simulink model "test_aero"  (R2014b)
settings: Solver=ode45  StartTime=0.0  StopTime=10.0  RelTol=1e-3
values from neighbouring files (symbols this model uses):
  TestInputs =     [unit_test_inputs.mat]
libraries: simulink x4, simulink_extras x2, csu_afm_aerodynamics_lib x1, util_frame_rotation_lib x1
settings Model: Creator=gnc  LastModifiedBy=mstewart
settings DebuggingCC: UnderspecifiedInitializationDetection=Classic  MergeDetectMultiDrivingBlocksExec=none  SolverPrmCheckMsg=none

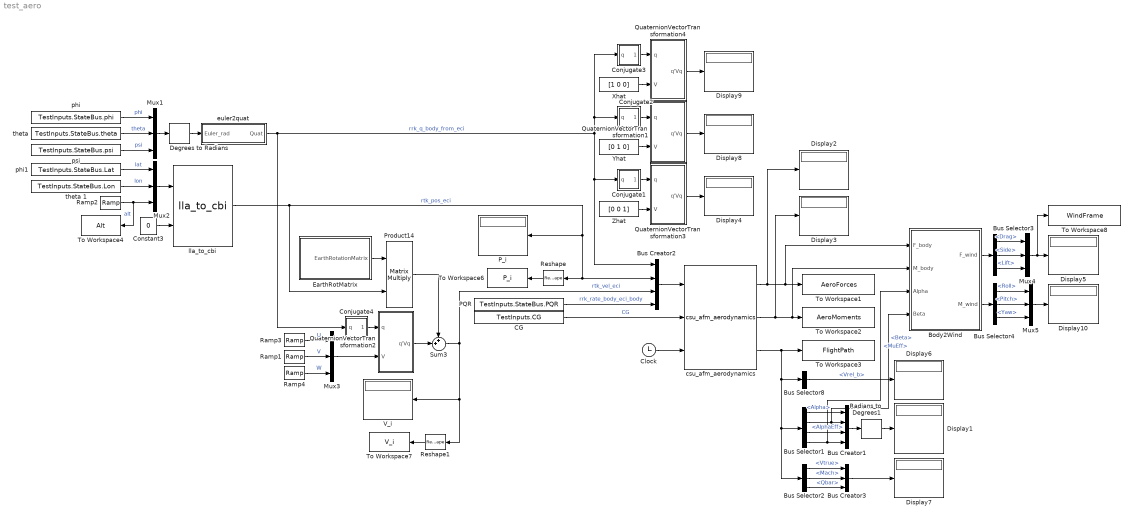
== system test_aero ==
  Body2Wind : Subsystem
  Bus Creator1 : BusCreator
  Bus Creator2 : BusCreator
  Bus Creator3 : BusCreator  Inputs=3
  Bus Selector1 : BusSelector  OutputSignals=Alpha,Beta,AlphaEff,MuEff
  Bus Selector2 : BusSelector  OutputSignals=Vtrue,Mach,Qbar
  Bus Selector3 : BusSelector  OutputSignals=Drag,Side,Lift
  Bus Selector4 : BusSelector  OutputSignals=Roll,Pitch,Yaw
  Bus Selector8 : BusSelector  OutputSignals=Vrel_b
  CG : Constant  Value=TestInputs.CG  VectorParams1D=off
  Clock : Clock
  Conjugate1 : Subsystem
  Conjugate2 : Subsystem
  Conjugate3 : Subsystem
  Conjugate4 : Subsystem
  Constant3 : Constant  Value=0
  Degrees to Radians : simulink_extras/Transformations/Degrees to Radians
  Display{1..10} (10 alike) : Display
  EarthRotMatrix : Subsystem
  Mux{1..5} (5 alike) : Mux  Inputs=3
  PQR : Constant  Value=TestInputs.StateBus.PQR  VectorParams1D=off
  P_i : Display
  Product14 : Product  Multiplication=Matrix(*)  SaturateOnIntegerOverflow=on  OutDataTypeStr=Inherit: Same as first input
  QuaternionVectorTransformation1 : Subsystem
  QuaternionVectorTransformation2 : Subsystem
  QuaternionVectorTransformation3 : Subsystem
  QuaternionVectorTransformation4 : Subsystem
  Radians to Degrees1 : simulink_extras/Transformations/Radians to Degrees
  Ramp1 : simulink/Sources/Ramp  slope=TestInputs.StateBus.Vdot  start=0  X0=TestInputs.StateBus.V
  Ramp2 : simulink/Sources/Ramp  slope=TestInputs.StateBus.AltDot  start=0  X0=TestInputs.StateBus.Alt
  Ramp3 : simulink/Sources/Ramp  slope=TestInputs.StateBus.Udot  start=0  X0=TestInputs.StateBus.U
  Ramp4 : simulink/Sources/Ramp  slope=TestInputs.StateBus.Wdot  start=0  X0=TestInputs.StateBus.W
  Reshape : Reshape
  Reshape1 : Reshape
  Sum3 : Sum  Inputs=++|
  To Workspace1 : ToWorkspace  VariableName=AeroForces  SaveFormat=Timeseries  SampleTime=-1
  To Workspace2 : ToWorkspace  VariableName=AeroMoments  SaveFormat=Timeseries  SampleTime=-1
  To Workspace3 : ToWorkspace  VariableName=FlightPath  SaveFormat=Timeseries  SampleTime=-1
  To Workspace4 : ToWorkspace  VariableName=Alt  SaveFormat=Timeseries  SampleTime=-1
  To Workspace6 : ToWorkspace  VariableName=P_i  SaveFormat=Timeseries  SampleTime=-1
  To Workspace7 : ToWorkspace  VariableName=V_i  SaveFormat=Timeseries  SampleTime=-1
  To Workspace8 : ToWorkspace  VariableName=WindFrame  SaveFormat=Timeseries  SampleTime=-1
  V_i : Display
  Xhat : Constant  Value=[1 0 0]
  Yhat : Constant  Value=[0 1 0]
  Zhat : Constant  Value=[0 0 1]
  csu_afm_aerodynamics : csu_afm_aerodynamics_lib/csu_afm_aerodynamics  SystemSampleTime=-1
  euler2quat : Subsystem
  lla_to_cbi : util_frame_rotation_lib/lla_to_cbi  a=6378137.0  flatten=1/298.257223563
  phi : Constant  Value=TestInputs.StateBus.phi  VectorParams1D=off
  phi1 : Constant  Value=TestInputs.StateBus.Lat  VectorParams1D=off
  psi : Constant  Value=TestInputs.StateBus.psi  VectorParams1D=off
  theta : Constant  Value=TestInputs.StateBus.theta  VectorParams1D=off
  theta 1 : Constant  Value=TestInputs.StateBus.Lon  VectorParams1D=off
  wires:
  Bus Creator2/1 -> csu_afm_aerodynamics/1
  Clock/1 -> csu_afm_aerodynamics/3
  CG/1 -> csu_afm_aerodynamics/2  "CG"
  csu_afm_aerodynamics/2 -> Display3/1, Body2Wind/2(M_body), To Workspace2/1
  csu_afm_aerodynamics/1 -> Display2/1, To Workspace1/1, Body2Wind/1(F_body)
  phi/1 -> Mux1/1  "phi"
  theta/1 -> Mux1/2  "theta"
  Mux1/1 -> Degrees to Radians/1
  Degrees to Radians/1 -> euler2quat/1(Euler_rad)
  psi/1 -> Mux1/3  "psi"
  euler2quat/1(Quat) -> Conjugate4/1(q), Bus Creator2/1, Conjugate1/1(q), Conjugate3/1(q), Conjugate2/1(q)  "rrk_q_body_from_eci"
  PQR/1 -> Bus Creator2/4  "rrk_rate_body_eci_body"
  Sum3/1 -> Reshape1/1, V_i/1, Bus Creator2/3  "rtk_vel_eci"
  lla_to_cbi/1 -> Product14/2, Bus Creator2/2, Reshape/1, P_i/1  "rtk_pos_eci"
  Constant3/1 -> lla_to_cbi/2
  Mux2/1 -> lla_to_cbi/1
  theta 1/1 -> Mux2/2  "lon"
  Ramp2/1 -> To Workspace4/1, Mux2/3  "alt"
  phi1/1 -> Mux2/1  "lat"
  csu_afm_aerodynamics/3 -> Bus Selector1/1, Bus Selector2/1, Bus Selector8/1, To Workspace3/1
  Zhat/1 -> QuaternionVectorTransformation3/2(V)
  QuaternionVectorTransformation3/1(q'Vq) -> Display4/1
  Conjugate1/1(q') -> QuaternionVectorTransformation3/1(q)
  Yhat/1 -> QuaternionVectorTransformation1/2(V)
  QuaternionVectorTransformation1/1(q'Vq) -> Display8/1
  Conjugate2/1(q') -> QuaternionVectorTransformation1/1(q)
  Xhat/1 -> QuaternionVectorTransformation4/2(V)
  QuaternionVectorTransformation4/1(q'Vq) -> Display9/1
  Conjugate3/1(q') -> QuaternionVectorTransformation4/1(q)
  Bus Selector8/1 -> Display6/1  "<Vrel_b>"
  Bus Selector1/4 -> Body2Wind/3(Alpha), Bus Creator1/4  "<MuEff>"
  Bus Selector1/3 -> Bus Creator1/3  "<AlphaEff>"
  Bus Selector1/2 -> Body2Wind/4(Beta), Bus Creator1/2  "<Beta>"
  Bus Selector1/1 -> Bus Creator1/1  "<Alpha>"
  Bus Creator3/1 -> Display7/1
  Ramp3/1 -> Mux3/1  "U"
  Ramp1/1 -> Mux3/2  "V"
  Mux3/1 -> QuaternionVectorTransformation2/2(V)
  Ramp4/1 -> Mux3/3  "W"
  Conjugate4/1(q') -> QuaternionVectorTransformation2/1(q)
  EarthRotMatrix/1(EarthRotationMatrix) -> Product14/1
  QuaternionVectorTransformation2/1(q'Vq) -> Sum3/2
  Product14/1 -> Sum3/1
  Reshape1/1 -> To Workspace7/1
  Reshape/1 -> To Workspace6/1
  Bus Creator1/1 -> Radians to Degrees1/1
  Radians to Degrees1/1 -> Display1/1
  Body2Wind/1(F_wind) -> Bus Selector3/1
  Mux4/1 -> To Workspace8/1, Display5/1
  Bus Selector3/1 -> Mux4/1  "<Drag>"
  Bus Selector3/2 -> Mux4/2  "<Side>"
  Bus Selector3/3 -> Mux4/3  "<Lift>"
  Bus Selector2/1 -> Bus Creator3/1  "<Vtrue>"
  Bus Selector2/2 -> Bus Creator3/2  "<Mach>"
  Bus Selector2/3 -> Bus Creator3/3  "<Qbar>"
  Body2Wind/2(M_wind) -> Bus Selector4/1
  Bus Selector4/1 -> Mux5/1  "<Roll>"
  Bus Selector4/2 -> Mux5/2  "<Pitch>"
  Bus Selector4/3 -> Mux5/3  "<Yaw>"
  Mux5/1 -> Display10/1

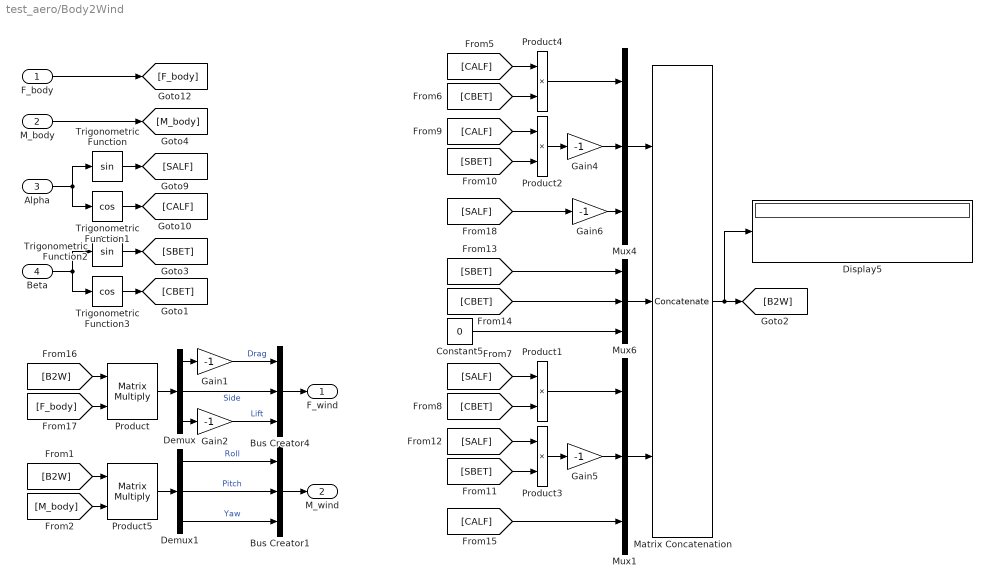
== system test_aero/Body2Wind ==
  F_body : Inport
  M_body : Inport  Port=2
  Alpha : Inport  Port=3
  Beta : Inport  Port=4
  Bus Creator1 : BusCreator  Inputs=3
  Bus Creator4 : BusCreator  Inputs=3
  Constant5 : Constant  Value=0
  Demux : Demux  Outputs=3
  Demux1 : Demux  Outputs=3
  Display5 : Display
  Gain{1..2,4..6} (5 alike) : Gain  Gain=-1  SaturateOnIntegerOverflow=on  OutDataTypeStr=Inherit: Same as input  ParamDataTypeStr=Inherit: Same as input
  Matrix Concatenation : Concatenate  NumInputs=3  Mode=Multidimensional array  ConcatenateDimension=2
  Mux1 : Mux  Inputs=3
  Mux4 : Mux  Inputs=3
  Mux6 : Mux  Inputs=3
  Product : Product  Multiplication=Matrix(*)  SaturateOnIntegerOverflow=on  OutDataTypeStr=Inherit: Same as first input
  Product{1..4} (4 alike) : Product  RndMeth=Zero
  Product5 : Product  Multiplication=Matrix(*)  SaturateOnIntegerOverflow=on  OutDataTypeStr=Inherit: Same as first input
  Trigonometric Function : Trigonometry
  Trigonometric Function1 : Trigonometry  Operator=cos
  Trigonometric Function2 : Trigonometry
  Trigonometric Function3 : Trigonometry  Operator=cos
  F_wind : Outport
  M_wind : Outport  Port=2
  wires:
  Trigonometric Function/1 -> [SALF]
  Trigonometric Function1/1 -> [CALF]
  Alpha/1 -> Trigonometric Function1/1, Trigonometric Function/1
  [B2W] -> Product/1
  [F_body] -> Product/2
  Product/1 -> Demux/1
  Demux/1 -> Gain1/1
  Demux/3 -> Gain2/1
  F_body/1 -> [F_body]
  Bus Creator4/1 -> F_wind/1
  Gain1/1 -> Bus Creator4/1  "Drag"
  Demux/2 -> Bus Creator4/2  "Side"
  Gain2/1 -> Bus Creator4/3  "Lift"
  Trigonometric Function2/1 -> [SBET]
  Trigonometric Function3/1 -> [CBET]
  Beta/1 -> Trigonometric Function3/1, Trigonometric Function2/1
  [CALF] -> Product4/1
  [CBET] -> Product4/2
  Product4/1 -> Mux4/1
  Matrix Concatenation/1 -> Display5/1, [B2W]
  Mux4/1 -> Matrix Concatenation/1
  [SALF] -> Product1/1
  [CBET] -> Product1/2
  [CALF] -> Product2/1
  [SBET] -> Product2/2
  Product2/1 -> Gain4/1
  [SALF] -> Gain6/1
  Mux6/1 -> Matrix Concatenation/2
  [SBET] -> Mux6/1
  Gain4/1 -> Mux4/2
  Gain6/1 -> Mux4/3
  Mux1/1 -> Matrix Concatenation/3
  Constant5/1 -> Mux6/3
  [CBET] -> Mux6/2
  Product1/1 -> Mux1/1
  [SALF] -> Product3/1
  [SBET] -> Product3/2
  Product3/1 -> Gain5/1
  Gain5/1 -> Mux1/2
  [CALF] -> Mux1/3
  [B2W] -> Product5/1
  [M_body] -> Product5/2
  Product5/1 -> Demux1/1
  Bus Creator1/1 -> M_wind/1
  Demux1/1 -> Bus Creator1/1  "Roll"
  Demux1/2 -> Bus Creator1/2  "Pitch"
  Demux1/3 -> Bus Creator1/3  "Yaw"
  M_body/1 -> [M_body]

== system test_aero/Conjugate1 ==
  q : Inport  PortDimensions=4
  Demux : Demux  Outputs=[3 1]
  Gain : Gain  Gain=-1  SaturateOnIntegerOverflow=on  OutDataTypeStr=Inherit: Same as input  ParamDataTypeStr=Inherit: Same as input
  Mux : Mux  Inputs=2
  q' : Outport  InitialOutput=0
  wires:
  q/1 -> Demux/1
  Demux/1 -> Gain/1  "[ q(1)  q(2)  q(3) ]"
  Gain/1 -> Mux/1
  Demux/2 -> Mux/2  "q(4)"
  Mux/1 -> q'/1

== system test_aero/Conjugate2 ==
  q : Inport  PortDimensions=4
  Demux : Demux  Outputs=[3 1]
  Gain : Gain  Gain=-1  SaturateOnIntegerOverflow=on  OutDataTypeStr=Inherit: Same as input  ParamDataTypeStr=Inherit: Same as input
  Mux : Mux  Inputs=2
  q' : Outport  InitialOutput=0
  wires:
  Mux/1 -> q'/1
  Demux/2 -> Mux/2  "q(4)"
  Gain/1 -> Mux/1
  Demux/1 -> Gain/1  "[ q(1)  q(2)  q(3) ]"
  q/1 -> Demux/1

== system test_aero/Conjugate3 ==
  q : Inport  PortDimensions=4
  Demux : Demux  Outputs=[3 1]
  Gain : Gain  Gain=-1  SaturateOnIntegerOverflow=on  OutDataTypeStr=Inherit: Same as input  ParamDataTypeStr=Inherit: Same as input
  Mux : Mux  Inputs=2
  q' : Outport  InitialOutput=0
  wires:
  Mux/1 -> q'/1
  Demux/2 -> Mux/2  "q(4)"
  Gain/1 -> Mux/1
  Demux/1 -> Gain/1  "[ q(1)  q(2)  q(3) ]"
  q/1 -> Demux/1

== system test_aero/Conjugate4 ==
  q : Inport  PortDimensions=4
  Demux : Demux  Outputs=[3 1]
  Gain : Gain  Gain=-1  SaturateOnIntegerOverflow=on  OutDataTypeStr=Inherit: Same as input  ParamDataTypeStr=Inherit: Same as input
  Mux : Mux  Inputs=2
  q' : Outport  InitialOutput=0
  wires:
  q/1 -> Demux/1
  Demux/1 -> Gain/1  "[ q(1)  q(2)  q(3) ]"
  Gain/1 -> Mux/1
  Demux/2 -> Mux/2  "q(4)"
  Mux/1 -> q'/1

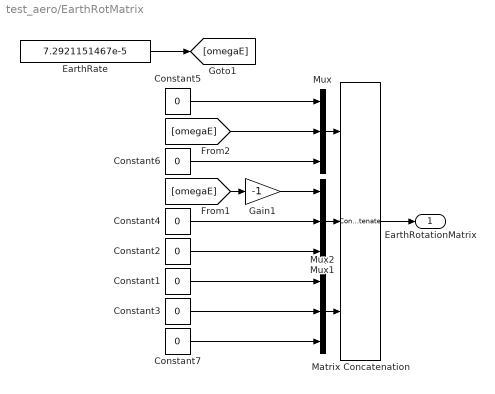
== system test_aero/EarthRotMatrix ==
  Constant{1..7} (7 alike) : Constant  Value=0
  EarthRate : Constant  Value=7.2921151467e-5
  Gain1 : Gain  Gain=-1  SaturateOnIntegerOverflow=on  OutDataTypeStr=Inherit: Same as input  ParamDataTypeStr=Inherit: Same as input
  Matrix Concatenation : Concatenate  NumInputs=3  Mode=Multidimensional array  ConcatenateDimension=2
  Mux : Mux  Inputs=3
  Mux1 : Mux  Inputs=3
  Mux2 : Mux  Inputs=3
  EarthRotationMatrix : Outport
  wires:
  [omegaE] -> Gain1/1
  Mux/1 -> Matrix Concatenation/1
  Mux1/1 -> Matrix Concatenation/2
  Gain1/1 -> Mux1/1
  Constant2/1 -> Mux1/3
  Constant1/1 -> Mux2/1
  Constant3/1 -> Mux2/2
  Constant7/1 -> Mux2/3
  Constant4/1 -> Mux1/2
  Constant6/1 -> Mux/3
  Constant5/1 -> Mux/1
  [omegaE] -> Mux/2
  EarthRate/1 -> [omegaE]
  Matrix Concatenation/1 -> EarthRotationMatrix/1
  Mux2/1 -> Matrix Concatenation/3

== system test_aero/QuaternionVectorTransformation1 ==
  q : Inport  PortDimensions=4
  V : Inport  Port=2  PortDimensions=3
  Constant : Constant  Value=0
  Mux : Mux  Inputs=2
  Quaternion Conjugate : Subsystem
  Quaternion Multiply : Subsystem
  Quaternion Multiply1 : Subsystem
  Selector : Selector  InputPortWidth=4  Indices=[1 2 3]
  q'Vq : Outport  InitialOutput=0
  wires:
  Quaternion Multiply/1(q1q2) -> Quaternion Multiply1/1(q1)
  Quaternion Conjugate/1(q') -> Quaternion Multiply/1(q1)
  Mux/1 -> Quaternion Multiply/2(q2)
  Quaternion Multiply1/1(q1q2) -> Selector/1
  q/1 -> Quaternion Conjugate/1(q), Quaternion Multiply1/2(q2)
  Constant/1 -> Mux/2
  V/1 -> Mux/1
  Selector/1 -> q'Vq/1

== system test_aero/QuaternionVectorTransformation2 ==
  q : Inport  PortDimensions=4
  V : Inport  Port=2  PortDimensions=3
  Constant : Constant  Value=0
  Mux : Mux  Inputs=2
  Quaternion Conjugate : Subsystem
  Quaternion Multiply : Subsystem
  Quaternion Multiply1 : Subsystem
  Selector : Selector  InputPortWidth=4  Indices=[1 2 3]
  q'Vq : Outport  InitialOutput=0
  wires:
  Selector/1 -> q'Vq/1
  V/1 -> Mux/1
  Constant/1 -> Mux/2
  q/1 -> Quaternion Multiply1/2(q2), Quaternion Conjugate/1(q)
  Quaternion Multiply1/1(q1q2) -> Selector/1
  Mux/1 -> Quaternion Multiply/2(q2)
  Quaternion Conjugate/1(q') -> Quaternion Multiply/1(q1)
  Quaternion Multiply/1(q1q2) -> Quaternion Multiply1/1(q1)

== system test_aero/QuaternionVectorTransformation3 ==
  q : Inport  PortDimensions=4
  V : Inport  Port=2  PortDimensions=3
  Constant : Constant  Value=0
  Mux : Mux  Inputs=2
  Quaternion Conjugate : Subsystem
  Quaternion Multiply : Subsystem
  Quaternion Multiply1 : Subsystem
  Selector : Selector  InputPortWidth=4  Indices=[1 2 3]
  q'Vq : Outport  InitialOutput=0
  wires:
  Selector/1 -> q'Vq/1
  V/1 -> Mux/1
  Constant/1 -> Mux/2
  q/1 -> Quaternion Multiply1/2(q2), Quaternion Conjugate/1(q)
  Quaternion Multiply1/1(q1q2) -> Selector/1
  Mux/1 -> Quaternion Multiply/2(q2)
  Quaternion Conjugate/1(q') -> Quaternion Multiply/1(q1)
  Quaternion Multiply/1(q1q2) -> Quaternion Multiply1/1(q1)

== system test_aero/QuaternionVectorTransformation4 ==
  q : Inport  PortDimensions=4
  V : Inport  Port=2  PortDimensions=3
  Constant : Constant  Value=0
  Mux : Mux  Inputs=2
  Quaternion Conjugate : Subsystem
  Quaternion Multiply : Subsystem
  Quaternion Multiply1 : Subsystem
  Selector : Selector  InputPortWidth=4  Indices=[1 2 3]
  q'Vq : Outport  InitialOutput=0
  wires:
  Quaternion Multiply/1(q1q2) -> Quaternion Multiply1/1(q1)
  Quaternion Conjugate/1(q') -> Quaternion Multiply/1(q1)
  Mux/1 -> Quaternion Multiply/2(q2)
  Quaternion Multiply1/1(q1q2) -> Selector/1
  q/1 -> Quaternion Conjugate/1(q), Quaternion Multiply1/2(q2)
  Constant/1 -> Mux/2
  V/1 -> Mux/1
  Selector/1 -> q'Vq/1

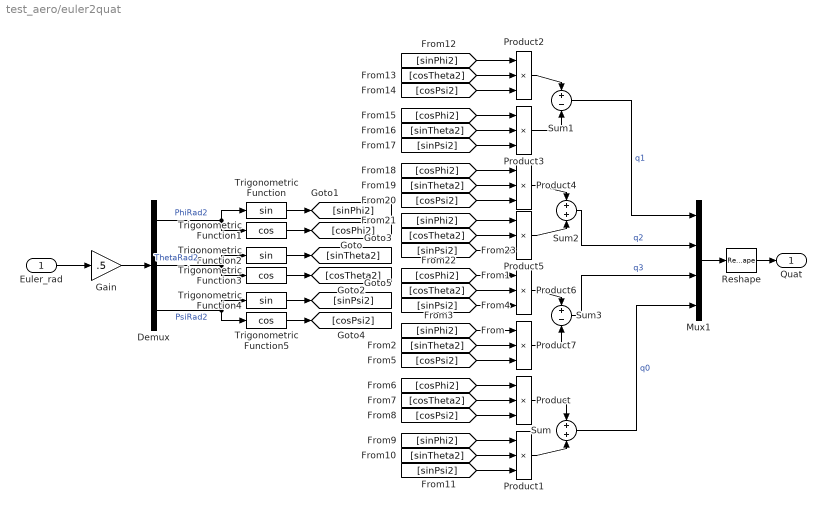
== system test_aero/euler2quat ==
  Euler_rad : Inport
  Demux : Demux  Outputs=3
  Gain : Gain  Gain=.5
  Mux1 : Mux
  Product{,1..7} (8 alike) : Product  Inputs=3  RndMeth=Zero
  Reshape : Reshape
  Sum : Sum  Inputs=+|+
  Sum1 : Sum  Inputs=+|-
  Sum2 : Sum  Inputs=+|+
  Sum3 : Sum  Inputs=+|-
  Trigonometric Function : Trigonometry
  Trigonometric Function1 : Trigonometry  Operator=cos
  Trigonometric Function2 : Trigonometry
  Trigonometric Function3 : Trigonometry  Operator=cos
  Trigonometric Function4 : Trigonometry
  Trigonometric Function5 : Trigonometry  Operator=cos
  Quat : Outport
  wires:
  Reshape/1 -> Quat/1
  Mux1/1 -> Reshape/1
  Euler_rad/1 -> Gain/1
  [cosPsi2] -> Product7/3
  [sinTheta2] -> Product7/2
  [sinPhi2] -> Product7/1
  [sinPsi2] -> Product6/3
  [cosTheta2] -> Product6/2
  [cosPhi2] -> Product6/1
  Product6/1 -> Sum3/1
  Product7/1 -> Sum3/2
  Product5/1 -> Sum2/2
  [sinPsi2] -> Product5/3
  [cosTheta2] -> Product5/2
  [sinPhi2] -> Product5/1
  Product4/1 -> Sum2/1
  [cosPsi2] -> Product4/3
  [sinTheta2] -> Product4/2
  [cosPhi2] -> Product4/1
  Product3/1 -> Sum1/2
  [sinPsi2] -> Product3/3
  [sinTheta2] -> Product3/2
  [cosPhi2] -> Product3/1
  Product2/1 -> Sum1/1
  [cosPsi2] -> Product2/3
  [cosTheta2] -> Product2/2
  [sinPhi2] -> Product2/1
  [sinPsi2] -> Product1/3
  [sinTheta2] -> Product1/2
  [sinPhi2] -> Product1/1
  Product1/1 -> Sum/2
  Product/1 -> Sum/1
  [cosPsi2] -> Product/3
  [cosTheta2] -> Product/2
  [cosPhi2] -> Product/1
  Trigonometric Function5/1 -> [cosPsi2]
  Trigonometric Function4/1 -> [sinPsi2]
  Trigonometric Function3/1 -> [cosTheta2]
  Trigonometric Function2/1 -> [sinTheta2]
  Trigonometric Function1/1 -> [cosPhi2]
  Trigonometric Function/1 -> [sinPhi2]
  Demux/3 -> Trigonometric Function5/1, Trigonometric Function4/1  "PsiRad2"
  Demux/2 -> Trigonometric Function3/1, Trigonometric Function2/1  "ThetaRad2"
  Demux/1 -> Trigonometric Function1/1, Trigonometric Function/1  "PhiRad2"
  Gain/1 -> Demux/1
  Sum1/1 -> Mux1/1  "q1"
  Sum2/1 -> Mux1/2  "q2"
  Sum3/1 -> Mux1/3  "q3"
  Sum/1 -> Mux1/4  "q0"

== system test_aero/QuaternionVectorTransformation1/Quaternion Conjugate ==
  q : Inport  PortDimensions=4
  Demux : Demux  Outputs=[3 1]
  Gain : Gain  Gain=-1  SaturateOnIntegerOverflow=on  OutDataTypeStr=Inherit: Same as input  ParamDataTypeStr=Inherit: Same as input
  Mux : Mux  Inputs=2
  q' : Outport  InitialOutput=0
  wires:
  Mux/1 -> q'/1
  Demux/2 -> Mux/2  "q(4)"
  Gain/1 -> Mux/1
  Demux/1 -> Gain/1  "[ q(1)  q(2)  q(3) ]"
  q/1 -> Demux/1

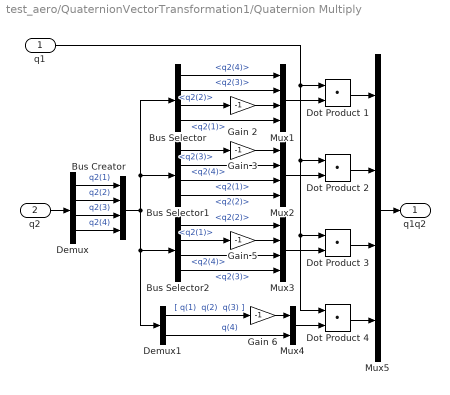
== system test_aero/QuaternionVectorTransformation1/Quaternion Multiply ==
  q1 : Inport  PortDimensions=4
  q2 : Inport  Port=2  PortDimensions=4
  Bus Creator : BusCreator
  Bus Selector : BusSelector  OutputSignals=q2(4),q2(3),q2(2),q2(1)
  Bus Selector1 : BusSelector  OutputSignals=q2(3),q2(4),q2(1),q2(2)
  Bus Selector2 : BusSelector  OutputSignals=q2(2),q2(1),q2(4),q2(3)
  Demux : Demux
  Demux1 : Demux  Outputs=[3 1]
  Dot Product {1..4} (4 alike) : DotProduct  InputSameDT=on  OutDataTypeStr=Inherit: Inherit via internal rule
  Gain {2..3,5..6} (4 alike) : Gain  Gain=-1  SaturateOnIntegerOverflow=on  OutDataTypeStr=Inherit: Same as input  ParamDataTypeStr=Inherit: Same as input
  Mux{1..3,5} (4 alike) : Mux
  Mux4 : Mux  Inputs=2
  q1q2 : Outport  InitialOutput=0
  wires:
  Demux/4 -> Bus Creator/4  "q2(4)"
  Demux/3 -> Bus Creator/3  "q2(3)"
  Demux/2 -> Bus Creator/2  "q2(2)"
  Demux/1 -> Bus Creator/1  "q2(1)"
  q2/1 -> Demux/1
  Bus Creator/1 -> Bus Selector1/1, Bus Selector/1, Bus Selector2/1, Demux1/1
  Dot Product 2/1 -> Mux5/2
  Mux5/1 -> q1q2/1
  Dot Product 4/1 -> Mux5/4
  Dot Product 3/1 -> Mux5/3
  Dot Product 1/1 -> Mux5/1
  q1/1 -> Dot Product 4/1, Dot Product 3/1, Dot Product 2/1, Dot Product 1/1
  Mux3/1 -> Dot Product 3/2
  Mux2/1 -> Dot Product 2/2
  Mux1/1 -> Dot Product 1/2
  Bus Selector2/3 -> Mux3/3  "<q2(4)>"
  Bus Selector1/2 -> Mux2/2  "<q2(4)>"
  Bus Selector/1 -> Mux1/1  "<q2(4)>"
  Bus Selector/2 -> Mux1/2  "<q2(3)>"
  Bus Selector/3 -> Gain 2/1  "<q2(2)>"
  Gain 2/1 -> Mux1/3
  Bus Selector/4 -> Mux1/4  "<q2(1)>"
  Bus Selector1/1 -> Gain 3/1  "<q2(3)>"
  Gain 3/1 -> Mux2/1
  Bus Selector1/3 -> Mux2/3  "<q2(1)>"
  Bus Selector1/4 -> Mux2/4  "<q2(2)>"
  Bus Selector2/2 -> Gain 5/1  "<q2(1)>"
  Gain 5/1 -> Mux3/2
  Bus Selector2/1 -> Mux3/1  "<q2(2)>"
  Bus Selector2/4 -> Mux3/4  "<q2(3)>"
  Mux4/1 -> Dot Product 4/2
  Demux1/1 -> Gain 6/1  "[ q(1)  q(2)  q(3) ]"
  Gain 6/1 -> Mux4/1
  Demux1/2 -> Mux4/2  "q(4)"

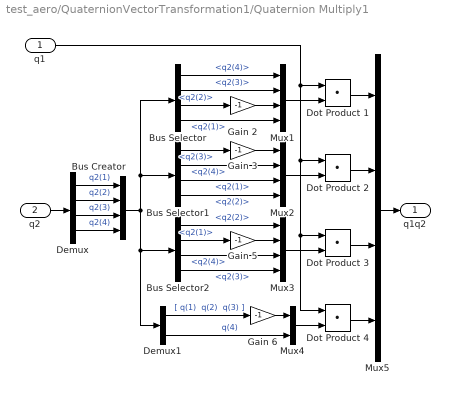
== system test_aero/QuaternionVectorTransformation1/Quaternion Multiply1 ==
  q1 : Inport  PortDimensions=4
  q2 : Inport  Port=2  PortDimensions=4
  Bus Creator : BusCreator
  Bus Selector : BusSelector  OutputSignals=q2(4),q2(3),q2(2),q2(1)
  Bus Selector1 : BusSelector  OutputSignals=q2(3),q2(4),q2(1),q2(2)
  Bus Selector2 : BusSelector  OutputSignals=q2(2),q2(1),q2(4),q2(3)
  Demux : Demux
  Demux1 : Demux  Outputs=[3 1]
  Dot Product {1..4} (4 alike) : DotProduct  InputSameDT=on  OutDataTypeStr=Inherit: Inherit via internal rule
  Gain {2..3,5..6} (4 alike) : Gain  Gain=-1  SaturateOnIntegerOverflow=on  OutDataTypeStr=Inherit: Same as input  ParamDataTypeStr=Inherit: Same as input
  Mux{1..3,5} (4 alike) : Mux
  Mux4 : Mux  Inputs=2
  q1q2 : Outport  InitialOutput=0
  wires:
  Demux/4 -> Bus Creator/4  "q2(4)"
  Demux/3 -> Bus Creator/3  "q2(3)"
  Demux/2 -> Bus Creator/2  "q2(2)"
  Demux/1 -> Bus Creator/1  "q2(1)"
  q2/1 -> Demux/1
  Bus Creator/1 -> Bus Selector1/1, Bus Selector/1, Bus Selector2/1, Demux1/1
  Dot Product 2/1 -> Mux5/2
  Mux5/1 -> q1q2/1
  Dot Product 4/1 -> Mux5/4
  Dot Product 3/1 -> Mux5/3
  Dot Product 1/1 -> Mux5/1
  q1/1 -> Dot Product 4/1, Dot Product 3/1, Dot Product 2/1, Dot Product 1/1
  Mux3/1 -> Dot Product 3/2
  Mux2/1 -> Dot Product 2/2
  Mux1/1 -> Dot Product 1/2
  Bus Selector2/3 -> Mux3/3  "<q2(4)>"
  Bus Selector1/2 -> Mux2/2  "<q2(4)>"
  Bus Selector/1 -> Mux1/1  "<q2(4)>"
  Bus Selector/2 -> Mux1/2  "<q2(3)>"
  Bus Selector/3 -> Gain 2/1  "<q2(2)>"
  Gain 2/1 -> Mux1/3
  Bus Selector/4 -> Mux1/4  "<q2(1)>"
  Bus Selector1/1 -> Gain 3/1  "<q2(3)>"
  Gain 3/1 -> Mux2/1
  Bus Selector1/3 -> Mux2/3  "<q2(1)>"
  Bus Selector1/4 -> Mux2/4  "<q2(2)>"
  Bus Selector2/2 -> Gain 5/1  "<q2(1)>"
  Gain 5/1 -> Mux3/2
  Bus Selector2/1 -> Mux3/1  "<q2(2)>"
  Bus Selector2/4 -> Mux3/4  "<q2(3)>"
  Mux4/1 -> Dot Product 4/2
  Demux1/1 -> Gain 6/1  "[ q(1)  q(2)  q(3) ]"
  Gain 6/1 -> Mux4/1
  Demux1/2 -> Mux4/2  "q(4)"

== system test_aero/QuaternionVectorTransformation2/Quaternion Conjugate ==
  q : Inport  PortDimensions=4
  Demux : Demux  Outputs=[3 1]
  Gain : Gain  Gain=-1  SaturateOnIntegerOverflow=on  OutDataTypeStr=Inherit: Same as input  ParamDataTypeStr=Inherit: Same as input
  Mux : Mux  Inputs=2
  q' : Outport  InitialOutput=0
  wires:
  q/1 -> Demux/1
  Demux/1 -> Gain/1  "[ q(1)  q(2)  q(3) ]"
  Gain/1 -> Mux/1
  Demux/2 -> Mux/2  "q(4)"
  Mux/1 -> q'/1

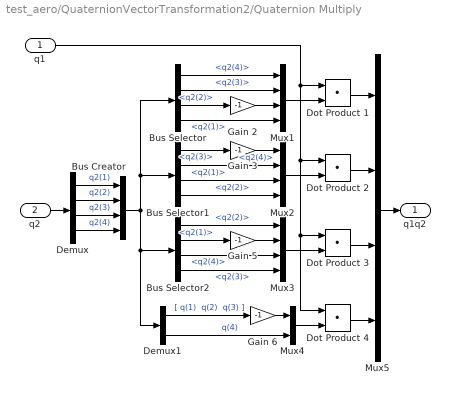
== system test_aero/QuaternionVectorTransformation2/Quaternion Multiply ==
  q1 : Inport  PortDimensions=4
  q2 : Inport  Port=2  PortDimensions=4
  Bus Creator : BusCreator
  Bus Selector : BusSelector  OutputSignals=q2(4),q2(3),q2(2),q2(1)
  Bus Selector1 : BusSelector  OutputSignals=q2(3),q2(4),q2(1),q2(2)
  Bus Selector2 : BusSelector  OutputSignals=q2(2),q2(1),q2(4),q2(3)
  Demux : Demux
  Demux1 : Demux  Outputs=[3 1]
  Dot Product {1..4} (4 alike) : DotProduct  InputSameDT=on  OutDataTypeStr=Inherit: Inherit via internal rule
  Gain {2..3,5..6} (4 alike) : Gain  Gain=-1  SaturateOnIntegerOverflow=on  OutDataTypeStr=Inherit: Same as input  ParamDataTypeStr=Inherit: Same as input
  Mux{1..3,5} (4 alike) : Mux
  Mux4 : Mux  Inputs=2
  q1q2 : Outport  InitialOutput=0
  wires:
  Demux1/2 -> Mux4/2  "q(4)"
  Gain 6/1 -> Mux4/1
  Demux1/1 -> Gain 6/1  "[ q(1)  q(2)  q(3) ]"
  Mux4/1 -> Dot Product 4/2
  Bus Selector2/4 -> Mux3/4  "<q2(3)>"
  Bus Selector2/1 -> Mux3/1  "<q2(2)>"
  Gain 5/1 -> Mux3/2
  Bus Selector2/2 -> Gain 5/1  "<q2(1)>"
  Bus Selector1/4 -> Mux2/4  "<q2(2)>"
  Bus Selector1/3 -> Mux2/3  "<q2(1)>"
  Gain 3/1 -> Mux2/1
  Bus Selector1/1 -> Gain 3/1  "<q2(3)>"
  Bus Selector/4 -> Mux1/4  "<q2(1)>"
  Gain 2/1 -> Mux1/3
  Bus Selector/3 -> Gain 2/1  "<q2(2)>"
  Bus Selector/2 -> Mux1/2  "<q2(3)>"
  Bus Selector/1 -> Mux1/1  "<q2(4)>"
  Bus Selector1/2 -> Mux2/2  "<q2(4)>"
  Bus Selector2/3 -> Mux3/3  "<q2(4)>"
  Mux1/1 -> Dot Product 1/2
  Mux2/1 -> Dot Product 2/2
  Mux3/1 -> Dot Product 3/2
  q1/1 -> Dot Product 1/1, Dot Product 2/1, Dot Product 3/1, Dot Product 4/1
  Dot Product 1/1 -> Mux5/1
  Dot Product 3/1 -> Mux5/3
  Dot Product 4/1 -> Mux5/4
  Mux5/1 -> q1q2/1
  Dot Product 2/1 -> Mux5/2
  Bus Creator/1 -> Demux1/1, Bus Selector2/1, Bus Selector/1, Bus Selector1/1
  q2/1 -> Demux/1
  Demux/1 -> Bus Creator/1  "q2(1)"
  Demux/2 -> Bus Creator/2  "q2(2)"
  Demux/3 -> Bus Creator/3  "q2(3)"
  Demux/4 -> Bus Creator/4  "q2(4)"

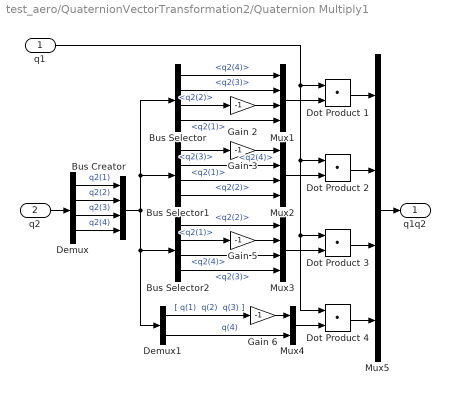
== system test_aero/QuaternionVectorTransformation2/Quaternion Multiply1 ==
  q1 : Inport  PortDimensions=4
  q2 : Inport  Port=2  PortDimensions=4
  Bus Creator : BusCreator
  Bus Selector : BusSelector  OutputSignals=q2(4),q2(3),q2(2),q2(1)
  Bus Selector1 : BusSelector  OutputSignals=q2(3),q2(4),q2(1),q2(2)
  Bus Selector2 : BusSelector  OutputSignals=q2(2),q2(1),q2(4),q2(3)
  Demux : Demux
  Demux1 : Demux  Outputs=[3 1]
  Dot Product {1..4} (4 alike) : DotProduct  InputSameDT=on  OutDataTypeStr=Inherit: Inherit via internal rule
  Gain {2..3,5..6} (4 alike) : Gain  Gain=-1  SaturateOnIntegerOverflow=on  OutDataTypeStr=Inherit: Same as input  ParamDataTypeStr=Inherit: Same as input
  Mux{1..3,5} (4 alike) : Mux
  Mux4 : Mux  Inputs=2
  q1q2 : Outport  InitialOutput=0
  wires:
  Demux1/2 -> Mux4/2  "q(4)"
  Gain 6/1 -> Mux4/1
  Demux1/1 -> Gain 6/1  "[ q(1)  q(2)  q(3) ]"
  Mux4/1 -> Dot Product 4/2
  Bus Selector2/4 -> Mux3/4  "<q2(3)>"
  Bus Selector2/1 -> Mux3/1  "<q2(2)>"
  Gain 5/1 -> Mux3/2
  Bus Selector2/2 -> Gain 5/1  "<q2(1)>"
  Bus Selector1/4 -> Mux2/4  "<q2(2)>"
  Bus Selector1/3 -> Mux2/3  "<q2(1)>"
  Gain 3/1 -> Mux2/1
  Bus Selector1/1 -> Gain 3/1  "<q2(3)>"
  Bus Selector/4 -> Mux1/4  "<q2(1)>"
  Gain 2/1 -> Mux1/3
  Bus Selector/3 -> Gain 2/1  "<q2(2)>"
  Bus Selector/2 -> Mux1/2  "<q2(3)>"
  Bus Selector/1 -> Mux1/1  "<q2(4)>"
  Bus Selector1/2 -> Mux2/2  "<q2(4)>"
  Bus Selector2/3 -> Mux3/3  "<q2(4)>"
  Mux1/1 -> Dot Product 1/2
  Mux2/1 -> Dot Product 2/2
  Mux3/1 -> Dot Product 3/2
  q1/1 -> Dot Product 1/1, Dot Product 2/1, Dot Product 3/1, Dot Product 4/1
  Dot Product 1/1 -> Mux5/1
  Dot Product 3/1 -> Mux5/3
  Dot Product 4/1 -> Mux5/4
  Mux5/1 -> q1q2/1
  Dot Product 2/1 -> Mux5/2
  Bus Creator/1 -> Demux1/1, Bus Selector2/1, Bus Selector/1, Bus Selector1/1
  q2/1 -> Demux/1
  Demux/1 -> Bus Creator/1  "q2(1)"
  Demux/2 -> Bus Creator/2  "q2(2)"
  Demux/3 -> Bus Creator/3  "q2(3)"
  Demux/4 -> Bus Creator/4  "q2(4)"

== system test_aero/QuaternionVectorTransformation3/Quaternion Conjugate ==
  q : Inport  PortDimensions=4
  Demux : Demux  Outputs=[3 1]
  Gain : Gain  Gain=-1  SaturateOnIntegerOverflow=on  OutDataTypeStr=Inherit: Same as input  ParamDataTypeStr=Inherit: Same as input
  Mux : Mux  Inputs=2
  q' : Outport  InitialOutput=0
  wires:
  q/1 -> Demux/1
  Demux/1 -> Gain/1  "[ q(1)  q(2)  q(3) ]"
  Gain/1 -> Mux/1
  Demux/2 -> Mux/2  "q(4)"
  Mux/1 -> q'/1

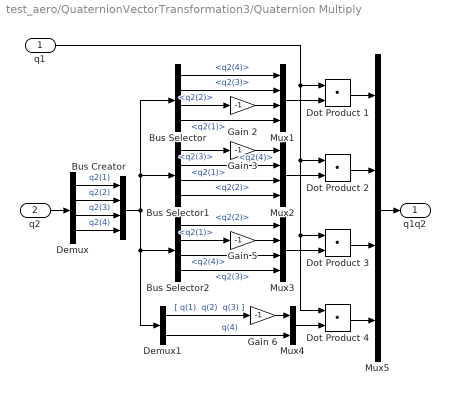
== system test_aero/QuaternionVectorTransformation3/Quaternion Multiply ==
  q1 : Inport  PortDimensions=4
  q2 : Inport  Port=2  PortDimensions=4
  Bus Creator : BusCreator
  Bus Selector : BusSelector  OutputSignals=q2(4),q2(3),q2(2),q2(1)
  Bus Selector1 : BusSelector  OutputSignals=q2(3),q2(4),q2(1),q2(2)
  Bus Selector2 : BusSelector  OutputSignals=q2(2),q2(1),q2(4),q2(3)
  Demux : Demux
  Demux1 : Demux  Outputs=[3 1]
  Dot Product {1..4} (4 alike) : DotProduct  InputSameDT=on  OutDataTypeStr=Inherit: Inherit via internal rule
  Gain {2..3,5..6} (4 alike) : Gain  Gain=-1  SaturateOnIntegerOverflow=on  OutDataTypeStr=Inherit: Same as input  ParamDataTypeStr=Inherit: Same as input
  Mux{1..3,5} (4 alike) : Mux
  Mux4 : Mux  Inputs=2
  q1q2 : Outport  InitialOutput=0
  wires:
  Demux1/2 -> Mux4/2  "q(4)"
  Gain 6/1 -> Mux4/1
  Demux1/1 -> Gain 6/1  "[ q(1)  q(2)  q(3) ]"
  Mux4/1 -> Dot Product 4/2
  Bus Selector2/4 -> Mux3/4  "<q2(3)>"
  Bus Selector2/1 -> Mux3/1  "<q2(2)>"
  Gain 5/1 -> Mux3/2
  Bus Selector2/2 -> Gain 5/1  "<q2(1)>"
  Bus Selector1/4 -> Mux2/4  "<q2(2)>"
  Bus Selector1/3 -> Mux2/3  "<q2(1)>"
  Gain 3/1 -> Mux2/1
  Bus Selector1/1 -> Gain 3/1  "<q2(3)>"
  Bus Selector/4 -> Mux1/4  "<q2(1)>"
  Gain 2/1 -> Mux1/3
  Bus Selector/3 -> Gain 2/1  "<q2(2)>"
  Bus Selector/2 -> Mux1/2  "<q2(3)>"
  Bus Selector/1 -> Mux1/1  "<q2(4)>"
  Bus Selector1/2 -> Mux2/2  "<q2(4)>"
  Bus Selector2/3 -> Mux3/3  "<q2(4)>"
  Mux1/1 -> Dot Product 1/2
  Mux2/1 -> Dot Product 2/2
  Mux3/1 -> Dot Product 3/2
  q1/1 -> Dot Product 1/1, Dot Product 2/1, Dot Product 3/1, Dot Product 4/1
  Dot Product 1/1 -> Mux5/1
  Dot Product 3/1 -> Mux5/3
  Dot Product 4/1 -> Mux5/4
  Mux5/1 -> q1q2/1
  Dot Product 2/1 -> Mux5/2
  Bus Creator/1 -> Demux1/1, Bus Selector2/1, Bus Selector/1, Bus Selector1/1
  q2/1 -> Demux/1
  Demux/1 -> Bus Creator/1  "q2(1)"
  Demux/2 -> Bus Creator/2  "q2(2)"
  Demux/3 -> Bus Creator/3  "q2(3)"
  Demux/4 -> Bus Creator/4  "q2(4)"

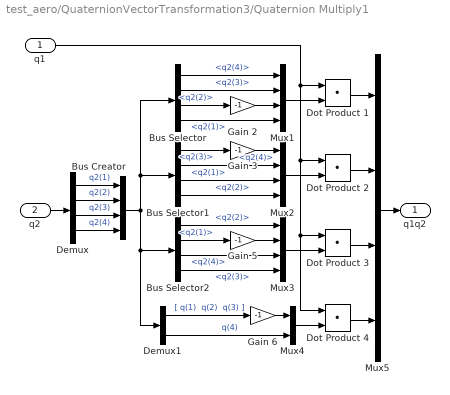
== system test_aero/QuaternionVectorTransformation3/Quaternion Multiply1 ==
  q1 : Inport  PortDimensions=4
  q2 : Inport  Port=2  PortDimensions=4
  Bus Creator : BusCreator
  Bus Selector : BusSelector  OutputSignals=q2(4),q2(3),q2(2),q2(1)
  Bus Selector1 : BusSelector  OutputSignals=q2(3),q2(4),q2(1),q2(2)
  Bus Selector2 : BusSelector  OutputSignals=q2(2),q2(1),q2(4),q2(3)
  Demux : Demux
  Demux1 : Demux  Outputs=[3 1]
  Dot Product {1..4} (4 alike) : DotProduct  InputSameDT=on  OutDataTypeStr=Inherit: Inherit via internal rule
  Gain {2..3,5..6} (4 alike) : Gain  Gain=-1  SaturateOnIntegerOverflow=on  OutDataTypeStr=Inherit: Same as input  ParamDataTypeStr=Inherit: Same as input
  Mux{1..3,5} (4 alike) : Mux
  Mux4 : Mux  Inputs=2
  q1q2 : Outport  InitialOutput=0
  wires:
  Demux1/2 -> Mux4/2  "q(4)"
  Gain 6/1 -> Mux4/1
  Demux1/1 -> Gain 6/1  "[ q(1)  q(2)  q(3) ]"
  Mux4/1 -> Dot Product 4/2
  Bus Selector2/4 -> Mux3/4  "<q2(3)>"
  Bus Selector2/1 -> Mux3/1  "<q2(2)>"
  Gain 5/1 -> Mux3/2
  Bus Selector2/2 -> Gain 5/1  "<q2(1)>"
  Bus Selector1/4 -> Mux2/4  "<q2(2)>"
  Bus Selector1/3 -> Mux2/3  "<q2(1)>"
  Gain 3/1 -> Mux2/1
  Bus Selector1/1 -> Gain 3/1  "<q2(3)>"
  Bus Selector/4 -> Mux1/4  "<q2(1)>"
  Gain 2/1 -> Mux1/3
  Bus Selector/3 -> Gain 2/1  "<q2(2)>"
  Bus Selector/2 -> Mux1/2  "<q2(3)>"
  Bus Selector/1 -> Mux1/1  "<q2(4)>"
  Bus Selector1/2 -> Mux2/2  "<q2(4)>"
  Bus Selector2/3 -> Mux3/3  "<q2(4)>"
  Mux1/1 -> Dot Product 1/2
  Mux2/1 -> Dot Product 2/2
  Mux3/1 -> Dot Product 3/2
  q1/1 -> Dot Product 1/1, Dot Product 2/1, Dot Product 3/1, Dot Product 4/1
  Dot Product 1/1 -> Mux5/1
  Dot Product 3/1 -> Mux5/3
  Dot Product 4/1 -> Mux5/4
  Mux5/1 -> q1q2/1
  Dot Product 2/1 -> Mux5/2
  Bus Creator/1 -> Demux1/1, Bus Selector2/1, Bus Selector/1, Bus Selector1/1
  q2/1 -> Demux/1
  Demux/1 -> Bus Creator/1  "q2(1)"
  Demux/2 -> Bus Creator/2  "q2(2)"
  Demux/3 -> Bus Creator/3  "q2(3)"
  Demux/4 -> Bus Creator/4  "q2(4)"

== system test_aero/QuaternionVectorTransformation4/Quaternion Conjugate ==
  q : Inport  PortDimensions=4
  Demux : Demux  Outputs=[3 1]
  Gain : Gain  Gain=-1  SaturateOnIntegerOverflow=on  OutDataTypeStr=Inherit: Same as input  ParamDataTypeStr=Inherit: Same as input
  Mux : Mux  Inputs=2
  q' : Outport  InitialOutput=0
  wires:
  Mux/1 -> q'/1
  Demux/2 -> Mux/2  "q(4)"
  Gain/1 -> Mux/1
  Demux/1 -> Gain/1  "[ q(1)  q(2)  q(3) ]"
  q/1 -> Demux/1

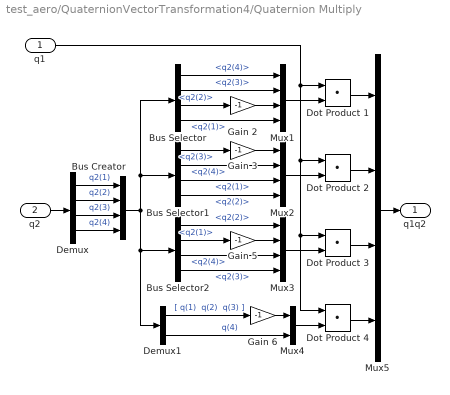
== system test_aero/QuaternionVectorTransformation4/Quaternion Multiply ==
  q1 : Inport  PortDimensions=4
  q2 : Inport  Port=2  PortDimensions=4
  Bus Creator : BusCreator
  Bus Selector : BusSelector  OutputSignals=q2(4),q2(3),q2(2),q2(1)
  Bus Selector1 : BusSelector  OutputSignals=q2(3),q2(4),q2(1),q2(2)
  Bus Selector2 : BusSelector  OutputSignals=q2(2),q2(1),q2(4),q2(3)
  Demux : Demux
  Demux1 : Demux  Outputs=[3 1]
  Dot Product {1..4} (4 alike) : DotProduct  InputSameDT=on  OutDataTypeStr=Inherit: Inherit via internal rule
  Gain {2..3,5..6} (4 alike) : Gain  Gain=-1  SaturateOnIntegerOverflow=on  OutDataTypeStr=Inherit: Same as input  ParamDataTypeStr=Inherit: Same as input
  Mux{1..3,5} (4 alike) : Mux
  Mux4 : Mux  Inputs=2
  q1q2 : Outport  InitialOutput=0
  wires:
  Demux/4 -> Bus Creator/4  "q2(4)"
  Demux/3 -> Bus Creator/3  "q2(3)"
  Demux/2 -> Bus Creator/2  "q2(2)"
  Demux/1 -> Bus Creator/1  "q2(1)"
  q2/1 -> Demux/1
  Bus Creator/1 -> Bus Selector1/1, Bus Selector/1, Bus Selector2/1, Demux1/1
  Dot Product 2/1 -> Mux5/2
  Mux5/1 -> q1q2/1
  Dot Product 4/1 -> Mux5/4
  Dot Product 3/1 -> Mux5/3
  Dot Product 1/1 -> Mux5/1
  q1/1 -> Dot Product 4/1, Dot Product 3/1, Dot Product 2/1, Dot Product 1/1
  Mux3/1 -> Dot Product 3/2
  Mux2/1 -> Dot Product 2/2
  Mux1/1 -> Dot Product 1/2
  Bus Selector2/3 -> Mux3/3  "<q2(4)>"
  Bus Selector1/2 -> Mux2/2  "<q2(4)>"
  Bus Selector/1 -> Mux1/1  "<q2(4)>"
  Bus Selector/2 -> Mux1/2  "<q2(3)>"
  Bus Selector/3 -> Gain 2/1  "<q2(2)>"
  Gain 2/1 -> Mux1/3
  Bus Selector/4 -> Mux1/4  "<q2(1)>"
  Bus Selector1/1 -> Gain 3/1  "<q2(3)>"
  Gain 3/1 -> Mux2/1
  Bus Selector1/3 -> Mux2/3  "<q2(1)>"
  Bus Selector1/4 -> Mux2/4  "<q2(2)>"
  Bus Selector2/2 -> Gain 5/1  "<q2(1)>"
  Gain 5/1 -> Mux3/2
  Bus Selector2/1 -> Mux3/1  "<q2(2)>"
  Bus Selector2/4 -> Mux3/4  "<q2(3)>"
  Mux4/1 -> Dot Product 4/2
  Demux1/1 -> Gain 6/1  "[ q(1)  q(2)  q(3) ]"
  Gain 6/1 -> Mux4/1
  Demux1/2 -> Mux4/2  "q(4)"

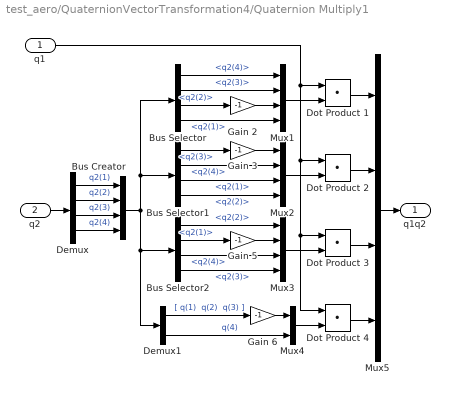
== system test_aero/QuaternionVectorTransformation4/Quaternion Multiply1 ==
  q1 : Inport  PortDimensions=4
  q2 : Inport  Port=2  PortDimensions=4
  Bus Creator : BusCreator
  Bus Selector : BusSelector  OutputSignals=q2(4),q2(3),q2(2),q2(1)
  Bus Selector1 : BusSelector  OutputSignals=q2(3),q2(4),q2(1),q2(2)
  Bus Selector2 : BusSelector  OutputSignals=q2(2),q2(1),q2(4),q2(3)
  Demux : Demux
  Demux1 : Demux  Outputs=[3 1]
  Dot Product {1..4} (4 alike) : DotProduct  InputSameDT=on  OutDataTypeStr=Inherit: Inherit via internal rule
  Gain {2..3,5..6} (4 alike) : Gain  Gain=-1  SaturateOnIntegerOverflow=on  OutDataTypeStr=Inherit: Same as input  ParamDataTypeStr=Inherit: Same as input
  Mux{1..3,5} (4 alike) : Mux
  Mux4 : Mux  Inputs=2
  q1q2 : Outport  InitialOutput=0
  wires:
  Demux/4 -> Bus Creator/4  "q2(4)"
  Demux/3 -> Bus Creator/3  "q2(3)"
  Demux/2 -> Bus Creator/2  "q2(2)"
  Demux/1 -> Bus Creator/1  "q2(1)"
  q2/1 -> Demux/1
  Bus Creator/1 -> Bus Selector1/1, Bus Selector/1, Bus Selector2/1, Demux1/1
  Dot Product 2/1 -> Mux5/2
  Mux5/1 -> q1q2/1
  Dot Product 4/1 -> Mux5/4
  Dot Product 3/1 -> Mux5/3
  Dot Product 1/1 -> Mux5/1
  q1/1 -> Dot Product 4/1, Dot Product 3/1, Dot Product 2/1, Dot Product 1/1
  Mux3/1 -> Dot Product 3/2
  Mux2/1 -> Dot Product 2/2
  Mux1/1 -> Dot Product 1/2
  Bus Selector2/3 -> Mux3/3  "<q2(4)>"
  Bus Selector1/2 -> Mux2/2  "<q2(4)>"
  Bus Selector/1 -> Mux1/1  "<q2(4)>"
  Bus Selector/2 -> Mux1/2  "<q2(3)>"
  Bus Selector/3 -> Gain 2/1  "<q2(2)>"
  Gain 2/1 -> Mux1/3
  Bus Selector/4 -> Mux1/4  "<q2(1)>"
  Bus Selector1/1 -> Gain 3/1  "<q2(3)>"
  Gain 3/1 -> Mux2/1
  Bus Selector1/3 -> Mux2/3  "<q2(1)>"
  Bus Selector1/4 -> Mux2/4  "<q2(2)>"
  Bus Selector2/2 -> Gain 5/1  "<q2(1)>"
  Gain 5/1 -> Mux3/2
  Bus Selector2/1 -> Mux3/1  "<q2(2)>"
  Bus Selector2/4 -> Mux3/4  "<q2(3)>"
  Mux4/1 -> Dot Product 4/2
  Demux1/1 -> Gain 6/1  "[ q(1)  q(2)  q(3) ]"
  Gain 6/1 -> Mux4/1
  Demux1/2 -> Mux4/2  "q(4)"
